simulink model "ephasor_sim_test"  (R2015a)
settings: Solver=ode4  StartTime=0.0  StopTime=6  FixedStep=Ts  RelTol=1e-3
PreLoadFcn:
  | Ts=0.1;
PostLoadFcn:
  | Ts=0.1;
InitFcn:
  | Ts=0.1;
StartFcn:
  | Ts=0.1;
libraries: opal_lib x2, rtlab x2, dspindex x1, rtlab_phasor x1
settings Model: Creator=Jaimie.Swartz  LastModifiedBy=Jaimie.Swartz
settings SolverCC: AlgebraicLoopSolver=LineSearch
settings DataIOCC: SignalLoggingSaveFormat=ModelDataLogs  SignalLogging=off  DSMLogging=off  VisualizeSimOutput=off
settings OptimizationCC: ExpressionDepthLimit=2147483647
settings DebuggingCC: UnderspecifiedInitializationDetection=Classic  MergeDetectMultiDrivingBlocksExec=none  SolverPrmCheckMsg=warning  FcnCallInpInsideContextMsg=EnableAllAsWarning  StateNameClashWarn=warning
settings GRTTargetCC: CombineOutputUpdateFcns=off  GRTInterface=on

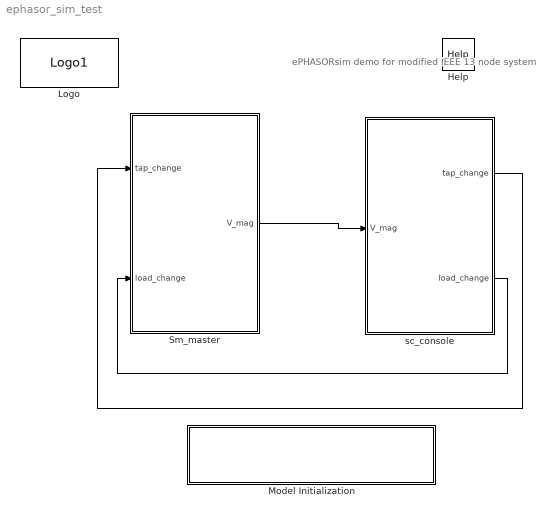
== system ephasor_sim_test ==
  note: ePHASORsim demo for
      | modified IEEE 13 node system
  Help : opal_lib/Help  docfile=../help/ePH_IEEE13.html
  Logo : opal_lib/Logo1  vide=[]
  Model Initialization : Subsystem  mask(Model Functions){InitFcnX=Ts=0.1;, prel=on, posl=on, inif=on, strf=on}
      mask prompts: InitFcnX "Initialisation"; prel "Preload Function"; posl "PostLoad Function"; inif "InitFcn"; strf "StartFcn"
      mask init:
      | currentBlock = gcb;
      | root = bdroot(currentBlock);
      | 
      | if ~strcmp(get_param(root,'BlockDiagramType'),'library')
      |     if prel==1
      |         set_param(root, 'PreLoadFcn', InitFcnX);
      |     else
      |         set_param(root, 'PreLoadFcn', '');
      |     end
      |     if inif==1
      |         set_param(root, 'InitFcn', InitFcnX);
      |     else
      |         set_param(root, 'InitFcn', '');
      |     end
      |     if strf==1
      |         set_param(root, 'StartFcn', InitFcnX);
      |     else
      |         set_param(root, 'StartFcn', '');
      |     end
      |     if posl==1
      |         set_param(root, 'PostLoadFcn', InitFcnX);
      |     else
      |         set_param(root, 'PostLoadFcn', '');
      |     end
      | end
      | 
      | pos = get_param(currentBlock, 'Position');
      | width = pos(3) - pos(1); height = pos(4) - pos(2);
      | txt = [ upper(root) '\n' '- InitFcn. . . . . '  get_param(root, 'InitFcn') ];
      settings: CopyFcn=set_param(gcb,'LinkStatus','none')
      mask Display: text(5, height*0.5, txt, 'horizontalAlignment', 'left', 'verticalAlignment', 'middle') ;
  Sm_master : Subsystem
  sc_console : Subsystem
  wires:
  Sm_master/1(V_mag) -> sc_console/1(V_mag)
  sc_console/1(tap_change) -> Sm_master/1(tap_change)
  sc_console/2(load_change) -> Sm_master/2(load_change)

== system ephasor_sim_test/Model Initialization ==

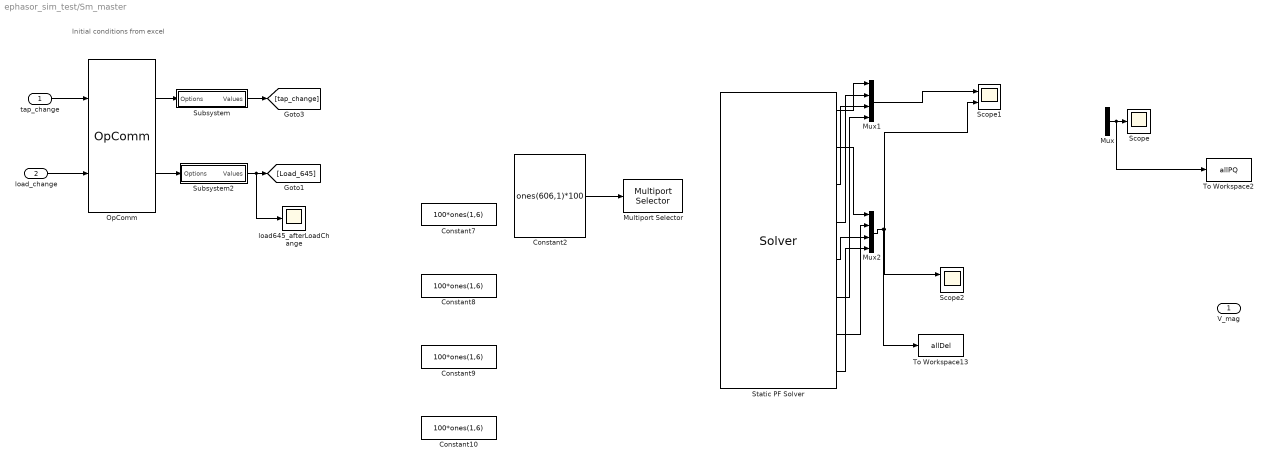
== system ephasor_sim_test/Sm_master ==
  note: Initial conditions from excel
  tap_change : Inport
  load_change : Inport  Port=2
  Constant{7..10} (4 alike) : Constant  Value=100*ones(1,6)
  Constant2 : Constant  Value=ones(606,1)*100
  Multiport Selector : dspindex/Multiport Selector  rowsOrCols=Rows  idxCellArray={ [1:254], [255:508], [509: 606]}  idxErrMode=Generate Error
  Mux : Mux  Inputs=3
  Mux1 : Mux
  Mux2 : Mux
  OpComm : rtlab/OpComm  nbport=2  groupe_acq=1  subsys_rate=0  st=0  Synchronization=on  Interpolation=on  Threshold=1.0  Missed_Data=off  Sim_Time=off  Samples=off  dynSigOut=off  from_console=1  warning_done=off  writeOpCommFile=off  Offset=off
  Scope : Scope
      settings: YMin=2225  YMax=2425
  Scope1 : Scope  NumInputPorts=2
      settings: YMin=-23.625~-5  YMax=2.625~5  SaveName=ScopeData2
  Scope2 : Scope  NumInputPorts=2
      settings: YMin=-23.625~-5  YMax=2.625~5  SaveName=ScopeData18
  Static PF Solver : rtlab_phasor/Solver  epname=System  extension=Excel  xls='PL0001_OPAL_working.xls'  raw='4992b.raw'  dyr='4992b.dyr'  cyme='ieee13.sxst'  powerfactory='network.dgs'  builtin=on  cyme_pf=''  cyme_unbalanced=on  lazy_netlist=on  capidir='CAPI'  fmudir='FMU'  capiprefix=capicomp_  fmuprefix=fmucomp_  logging=off  sim_mode=Dynamic simulation only (without power-flow)  pf_max_it=100  pf_tol_v=0.00000001  pf_flat_start=off  pf_smart_start=on  pf_export=on  np=1  exporty=off  dt=Ts  optim_threads=off  perflog_on=off  script_activate_postinit=off  script_postinit_name='python_integration_13NFbal.py'
  Subsystem : Subsystem
  Subsystem2 : Subsystem
  To Workspace13 : ToWorkspace  VariableName=allDel  SampleTime=-1
  To Workspace2 : ToWorkspace  VariableName=allPQ  SampleTime=-1
      settings: Save2DSignal=2-D array (concatenate along first dimension)
  load645_afterLoadChange : Scope
      settings: ShowLegends=on  YMin=0.94469  YMax=1.0518  SaveName=ScopeData17
  V_mag : Outport
  wires:
  tap_change/1 -> OpComm/1
  load_change/1 -> OpComm/2
  OpComm/1 -> Subsystem/1(Options)
  OpComm/2 -> Subsystem2/1(Options)
  Subsystem/1(Values) -> [tap_change]
  Subsystem2/1(Values) -> load645_afterLoadChange/1, [Load_645]
  ? -> V_mag/1
  Mux/1 -> To Workspace2/1, Scope/1
  Mux1/1 -> Scope1/1
  Mux2/1 -> To Workspace13/1, Scope1/2, Scope2/1
  Static PF Solver/2 -> Mux2/1
  Static PF Solver/7 -> Mux2/2
  Static PF Solver/5 -> Mux2/3
  Static PF Solver/8 -> Mux2/4
  Static PF Solver/1 -> Mux1/1
  Static PF Solver/4 -> Mux1/2
  Static PF Solver/3 -> Mux1/3
  Static PF Solver/6 -> Mux1/4
  Constant2/1 -> Multiport Selector/1

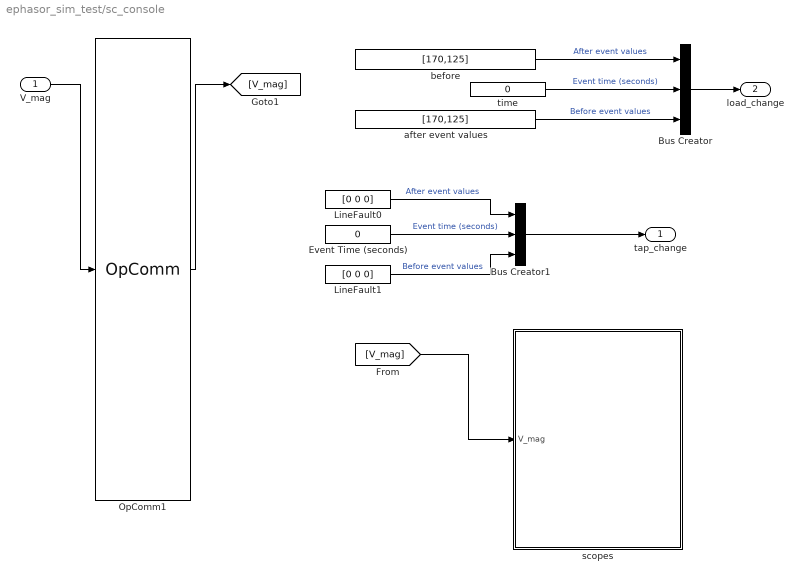
== system ephasor_sim_test/sc_console ==
  V_mag : Inport
  Bus Creator : BusCreator  Inputs=3
  Bus Creator1 : BusCreator  Inputs=3
  Event Time (seconds) : Constant  Value=0
  LineFault0 : Constant  Value=[0 0 0]
  LineFault1 : Constant  Value=[0 0 0]
  OpComm1 : rtlab/OpComm  nbport=1  groupe_acq=1  subsys_rate=0  st=0  Synchronization=on  Interpolation=on  Threshold=1.0  Missed_Data=off  Sim_Time=off  Samples=off  dynSigOut=off  from_console=0  warning_done=off  writeOpCommFile=off  Offset=off
  after event values : Constant  Value=[170,125]
  before : Constant  Value=[170,125]
  scopes : Subsystem
  time : Constant  Value=0
  tap_change : Outport
  load_change : Outport  Port=2
  wires:
  V_mag/1 -> OpComm1/1
  OpComm1/1 -> [V_mag]
  time/1 -> Bus Creator/2  "Event time (seconds)"
  Bus Creator/1 -> load_change/1
  LineFault0/1 -> Bus Creator1/1  "After event values"
  LineFault1/1 -> Bus Creator1/3  "Before event values"
  Event Time (seconds)/1 -> Bus Creator1/2  "Event time (seconds)"
  Bus Creator1/1 -> tap_change/1
  before/1 -> Bus Creator/1  "After event values"
  after event values/1 -> Bus Creator/3  "Before event values"
  [V_mag] -> scopes/1(V_mag)

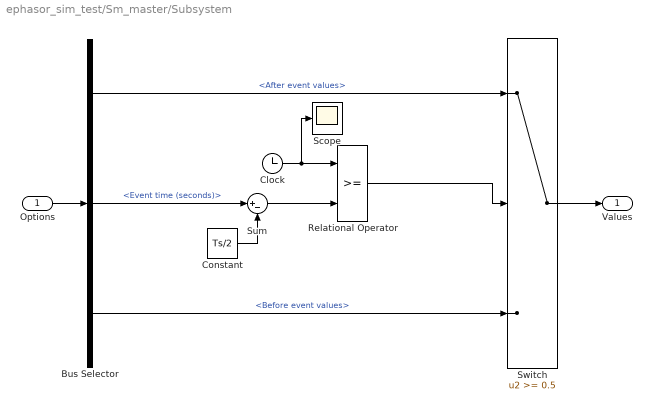
== system ephasor_sim_test/Sm_master/Subsystem ==
  Options : Inport
  Bus Selector : BusSelector  OutputSignals=After event values,Event time (seconds),Before event values
  Clock : Clock
  Constant : Constant  Value=Ts/2
  Relational Operator : RelationalOperator  OutDataTypeStr=boolean
  Scope : Scope
  Sum : Sum  Inputs=|+-
  Switch : Switch  Threshold=0.5
  Values : Outport
  wires:
  Clock/1 -> Scope/1, Relational Operator/1
  Constant/1 -> Sum/2
  Sum/1 -> Relational Operator/2
  Bus Selector/2 -> Sum/1  "<Event time (seconds)>"
  Relational Operator/1 -> Switch/2
  Bus Selector/3 -> Switch/3  "<Before event values>"
  Bus Selector/1 -> Switch/1  "<After event values>"
  Switch/1 -> Values/1
  Options/1 -> Bus Selector/1

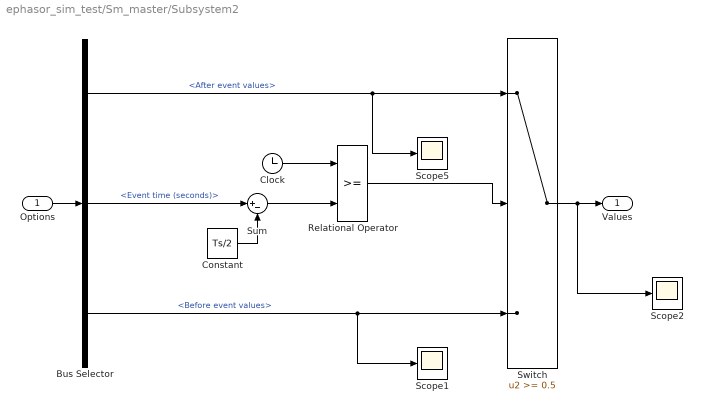
== system ephasor_sim_test/Sm_master/Subsystem2 ==
  Options : Inport
  Bus Selector : BusSelector  OutputSignals=After event values,Event time (seconds),Before event values
  Clock : Clock
  Constant : Constant  Value=Ts/2
  Relational Operator : RelationalOperator  OutDataTypeStr=boolean
  Scope1 : Scope
      settings: SaveName=ScopeData14
  Scope2 : Scope
      settings: SaveName=ScopeData15
  Scope5 : Scope
      settings: SaveName=ScopeData13
  Sum : Sum  Inputs=|+-
  Switch : Switch  Threshold=0.5
  Values : Outport
  wires:
  Clock/1 -> Relational Operator/1
  Constant/1 -> Sum/2
  Sum/1 -> Relational Operator/2
  Bus Selector/2 -> Sum/1  "<Event time (seconds)>"
  Relational Operator/1 -> Switch/2
  Bus Selector/3 -> Switch/3, Scope1/1  "<Before event values>"
  Bus Selector/1 -> Switch/1, Scope5/1  "<After event values>"
  Switch/1 -> Values/1, Scope2/1
  Options/1 -> Bus Selector/1

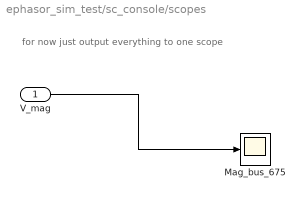
== system ephasor_sim_test/sc_console/scopes ==
  note: for now just output everything to one scope
  V_mag : Inport
  Mag_bus_675 : Scope
      settings: YMin=0.92  YMax=1.07  SaveName=ScopeData6
  wires:
  V_mag/1 -> Mag_bus_675/1
